simulink model "costas"  (Simulink 5.0)
settings: Solver=ode45  StartTime=0.0  StopTime=1  RelTol=1e-3
libraries: dsparch4 x3, commcontsrc2 x2, dspsigops x2, commdigbbndpm2 x1, commrandsrc2 x1
settings Model: LastModifiedBy=Daiming Qu

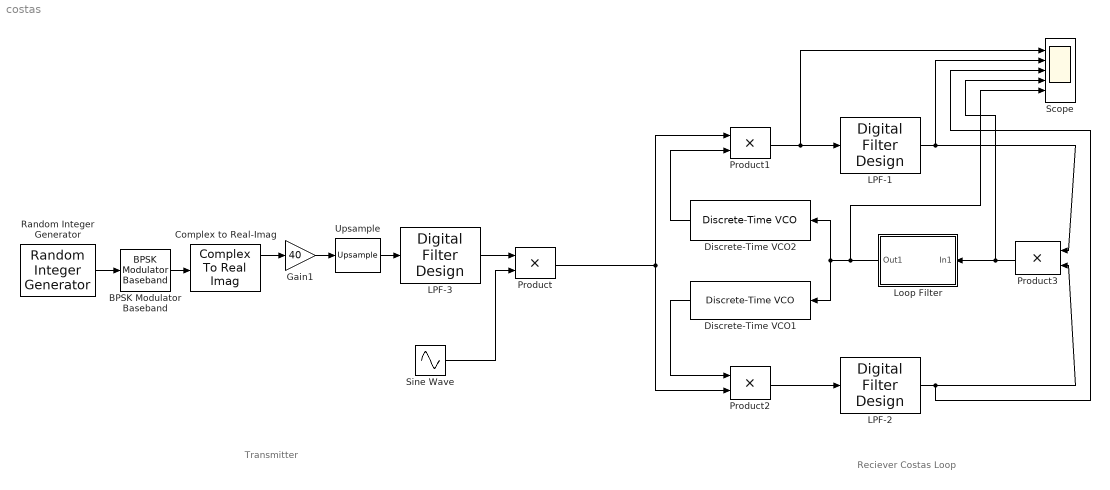
== system costas ==
  note: Transmitter
  note: Reciever
      | Costas Loop
  BPSK Modulator Baseband : commdigbbndpm2/BPSK Modulator Baseband  Ph=0  numSamp=1
  Complex to Real-Imag : ComplexToRealImag
  Discrete-Time VCO1 : commcontsrc2/Discrete-Time VCO  Orientation=left  Ac=1  Fc=1000  Kc=1  Ph=pi/2  ts=1/10000
  Discrete-Time VCO2 : commcontsrc2/Discrete-Time VCO  Orientation=left  Ac=1  Fc=1000  Kc=1  Ph=0  ts=1/10000
  Gain1 : Gain  Gain=40  SaturateOnIntegerOverflow=on
  LPF-1 : dsparch4/Digital Filter Design
  LPF-2 : dsparch4/Digital Filter Design
  LPF-3 : dsparch4/Digital Filter Design
  Loop Filter : Subsystem  Orientation=left
  Product : Product  SaturateOnIntegerOverflow=on
  Product1 : Product  SaturateOnIntegerOverflow=on
  Product2 : Product  SaturateOnIntegerOverflow=on
  Product3 : Product  Orientation=left  SaturateOnIntegerOverflow=on
  Random Integer Generator : commrandsrc2/Random Integer Generator  mul=2  seed=37  Ts=1/250  frameBased=off  sampPerFrame=1  orient=off
  Scope : Scope  NumInputPorts=5
      settings: YMin=-1.5~-5~-1~0~7.5  YMax=1.5~5~1~2~30  MaxDataPoints=10000
  Sine Wave : Sin  Frequency=1001*2*pi  Phase=pi/2  Samples=1000  SampleTime=1/10000
  Upsample : dspsigops/Upsample  N=40  phase=0  ic=0  mode=Maintain input frame size
  wires:
  Discrete-Time VCO2/1 -> Product1/2
  Product/1 -> Product2/2, Product1/1
  Product2/1 -> LPF-2/1
  Product1/1 -> LPF-1/1, Scope/1
  LPF-1/1 -> Scope/2, Product3/1
  Product3/1 -> Scope/4, Loop Filter/1(In1)
  Random Integer Generator/1 -> BPSK Modulator Baseband/1
  Sine Wave/1 -> Product/2
  Discrete-Time VCO1/1 -> Product2/1
  Loop Filter/1(Out1) -> Discrete-Time VCO2/1, Discrete-Time VCO1/1, Scope/5
  BPSK Modulator Baseband/1 -> Complex to Real-Imag/1
  Upsample/1 -> LPF-3/1
  LPF-3/1 -> Product/1
  LPF-2/1 -> Product3/2, Scope/3
  Complex to Real-Imag/1 -> Gain1/1
  Gain1/1 -> Upsample/1

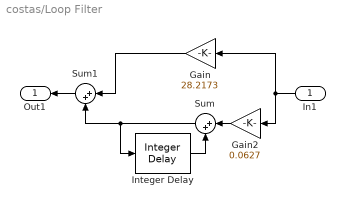
== system costas/Loop Filter ==
  In1 : Inport  Orientation=left
  Gain : Gain  Orientation=left  Gain=28.2173  SaturateOnIntegerOverflow=on
  Gain2 : Gain  Orientation=left  Gain=0.0627  SaturateOnIntegerOverflow=on
  Integer Delay : dspsigops/Integer Delay  delay=1  ic=0  reset_popup=None
  Sum : Sum  Orientation=left  Inputs=|++  SaturateOnIntegerOverflow=on
  Sum1 : Sum  Orientation=left  Inputs=|++  SaturateOnIntegerOverflow=on
  Out1 : Outport  Orientation=left
  wires:
  Gain2/1 -> Sum/1
  Gain/1 -> Sum1/1
  Sum/1 -> Integer Delay/1, Sum1/2
  Integer Delay/1 -> Sum/2
  In1/1 -> Gain2/1, Gain/1
  Sum1/1 -> Out1/1
